simulink model "RADTRANS001"  (R2020b)
(part 2 of 6)

  Трансформатор_110_6_Район_{1..5} (5 alike) : powerlib/Elements/Three-Phase Transformer (Two Windings)  Winding1Connection=Yg  Winding2Connection=Yg  CoreType=Three single-phase transformers  SetSaturation=off  Hysteresis=off  DataFile='hysteresis'  SetInitialFlux=off  Measurements=None  UNITS=pu  NominalPower=[Tr_110_6_Sn_VA, Sys_f_Hz]  Winding1=[Tr_110_6_V_HV_kV*1e3, Tr_110_6_R_pu, Tr_110_6_L_pu]  Winding2=[Tr_110_6_V_LV_kV*1e3, Tr_110_6_R_pu, Tr_110_6_L_pu]  Rm=500  Lm=500  L0=0.5  Saturation=[ 0,0 ; 0.0024,1.2 ; 1.0,1.52 ]  InitialFluxes=[ 0.8 , -0.8 , 0.7 ]  BreakLoop=off  DiscreteSolver=Trapezoidal iterative  DataType=off  TransfoNumber=1
  Трансформатор_Город_1_{1..4} (4 alike) : powerlib/Elements/Three-Phase Transformer (Two Windings)  Winding1Connection=Yg  Winding2Connection=Yg  CoreType=Three single-phase transformers  SetSaturation=off  Hysteresis=off  DataFile='hysteresis'  SetInitialFlux=off  Measurements=None  UNITS=pu  NominalPower=[Tr_6_04_Sn_VA, Sys_f_Hz]  Winding1=[Tr_6_04_V_HV_kV*1e3, Tr_6_04_R_pu, Tr_6_04_L_pu]  Winding2=[Tr_6_04_V_LV_kV*1e3, Tr_6_04_R_pu, Tr_6_04_L_pu]  Rm=500  Lm=500  L0=0.5  Saturation=[ 0,0 ; 0.0024,1.2 ; 1.0,1.52 ]  InitialFluxes=[ 0.8 , -0.8 , 0.7 ]  BreakLoop=off  DiscreteSolver=Trapezoidal iterative  DataType=off  TransfoNumber=1
  Трансформатор_Город_2_{1..4} (4 alike) : powerlib/Elements/Three-Phase Transformer (Two Windings)  Winding1Connection=Yg  Winding2Connection=Yg  CoreType=Three single-phase transformers  SetSaturation=off  Hysteresis=off  DataFile='hysteresis'  SetInitialFlux=off  Measurements=None  UNITS=pu  NominalPower=[Tr_6_04_Sn_VA, Sys_f_Hz]  Winding1=[Tr_6_04_V_HV_kV*1e3, Tr_6_04_R_pu, Tr_6_04_L_pu]  Winding2=[Tr_6_04_V_LV_kV*1e3, Tr_6_04_R_pu, Tr_6_04_L_pu]  Rm=500  Lm=500  L0=0.5  Saturation=[ 0,0 ; 0.0024,1.2 ; 1.0,1.52 ]  InitialFluxes=[ 0.8 , -0.8 , 0.7 ]  BreakLoop=off  DiscreteSolver=Trapezoidal iterative  DataType=off  TransfoNumber=1
  Трансформатор_Город_3_{1..4} (4 alike) : powerlib/Elements/Three-Phase Transformer (Two Windings)  Winding1Connection=Yg  Winding2Connection=Yg  CoreType=Three single-phase transformers  SetSaturation=off  Hysteresis=off  DataFile='hysteresis'  SetInitialFlux=off  Measurements=None  UNITS=pu  NominalPower=[Tr_6_04_Sn_VA, Sys_f_Hz]  Winding1=[Tr_6_04_V_HV_kV*1e3, Tr_6_04_R_pu, Tr_6_04_L_pu]  Winding2=[Tr_6_04_V_LV_kV*1e3, Tr_6_04_R_pu, Tr_6_04_L_pu]  Rm=500  Lm=500  L0=0.5  Saturation=[ 0,0 ; 0.0024,1.2 ; 1.0,1.52 ]  InitialFluxes=[ 0.8 , -0.8 , 0.7 ]  BreakLoop=off  DiscreteSolver=Trapezoidal iterative  DataType=off  TransfoNumber=1
  Трансформатор_Город_4_{1..4} (4 alike) : powerlib/Elements/Three-Phase Transformer (Two Windings)  Winding1Connection=Yg  Winding2Connection=Yg  CoreType=Three single-phase transformers  SetSaturation=off  Hysteresis=off  DataFile='hysteresis'  SetInitialFlux=off  Measurements=None  UNITS=pu  NominalPower=[Tr_6_04_Sn_VA, Sys_f_Hz]  Winding1=[Tr_6_04_V_HV_kV*1e3, Tr_6_04_R_pu, Tr_6_04_L_pu]  Winding2=[Tr_6_04_V_LV_kV*1e3, Tr_6_04_R_pu, Tr_6_04_L_pu]  Rm=500  Lm=500  L0=0.5  Saturation=[ 0,0 ; 0.0024,1.2 ; 1.0,1.52 ]  InitialFluxes=[ 0.8 , -0.8 , 0.7 ]  BreakLoop=off  DiscreteSolver=Trapezoidal iterative  DataType=off  TransfoNumber=1
  Трансформатор_Город_5_{1..4} (4 alike) : powerlib/Elements/Three-Phase Transformer (Two Windings)  Winding1Connection=Yg  Winding2Connection=Yg  CoreType=Three single-phase transformers  SetSaturation=off  Hysteresis=off  DataFile='hysteresis'  SetInitialFlux=off  Measurements=None  UNITS=pu  NominalPower=[Tr_6_04_Sn_VA, Sys_f_Hz]  Winding1=[Tr_6_04_V_HV_kV*1e3, Tr_6_04_R_pu, Tr_6_04_L_pu]  Winding2=[Tr_6_04_V_LV_kV*1e3, Tr_6_04_R_pu, Tr_6_04_L_pu]  Rm=500  Lm=500  L0=0.5  Saturation=[ 0,0 ; 0.0024,1.2 ; 1.0,1.52 ]  InitialFluxes=[ 0.8 , -0.8 , 0.7 ]  BreakLoop=off  DiscreteSolver=Trapezoidal iterative  DataType=off  TransfoNumber=1
  Трансформатор_Завод_1_1 : powerlib/Elements/Three-Phase Transformer (Two Windings)  Winding1Connection=Yg  Winding2Connection=Yg  CoreType=Three single-phase transformers  SetSaturation=off  Hysteresis=off  DataFile='hysteresis'  SetInitialFlux=off  Measurements=None  UNITS=pu  NominalPower=[Tr_35_04_Sn_VA, Sys_f_Hz]  Winding1=[Tr_35_04_V_HV_kV*1e3, Tr_35_04_R_pu, Tr_35_04_L_pu]  Winding2=[Tr_35_04_V_LV_kV*1e3, Tr_35_04_R_pu, Tr_35_04_L_pu]  Rm=500  Lm=500  L0=0.5  Saturation=[ 0,0 ; 0.0024,1.2 ; 1.0,1.52 ]  InitialFluxes=[ 0.8 , -0.8 , 0.7 ]  BreakLoop=off  DiscreteSolver=Trapezoidal iterative  DataType=off  TransfoNumber=1
  Трансформатор_Завод_1_2 : powerlib/Elements/Three-Phase Transformer (Two Windings)  Winding1Connection=Yg  Winding2Connection=Yg  CoreType=Three single-phase transformers  SetSaturation=off  Hysteresis=off  DataFile='hysteresis'  SetInitialFlux=off  Measurements=None  UNITS=pu  NominalPower=[Tr_35_04_Sn_VA, Sys_f_Hz]  Winding1=[Tr_35_04_V_HV_kV*1e3, Tr_35_04_R_pu, Tr_35_04_L_pu]  Winding2=[Tr_35_04_V_LV_kV*1e3, Tr_35_04_R_pu, Tr_35_04_L_pu]  Rm=500  Lm=500  L0=0.5  Saturation=[ 0,0 ; 0.0024,1.2 ; 1.0,1.52 ]  InitialFluxes=[ 0.8 , -0.8 , 0.7 ]  BreakLoop=off  DiscreteSolver=Trapezoidal iterative  DataType=off  TransfoNumber=1
  Трансформатор_Завод_2_1 : powerlib/Elements/Three-Phase Transformer (Two Windings)  Winding1Connection=Yg  Winding2Connection=Yg  CoreType=Three single-phase transformers  SetSaturation=off  Hysteresis=off  DataFile='hysteresis'  SetInitialFlux=off  Measurements=None  UNITS=pu  NominalPower=[Tr_35_04_Sn_VA, Sys_f_Hz]  Winding1=[Tr_35_04_V_HV_kV*1e3, Tr_35_04_R_pu, Tr_35_04_L_pu]  Winding2=[Tr_35_04_V_LV_kV*1e3, Tr_35_04_R_pu, Tr_35_04_L_pu]  Rm=500  Lm=500  L0=0.5  Saturation=[ 0,0 ; 0.0024,1.2 ; 1.0,1.52 ]  InitialFluxes=[ 0.8 , -0.8 , 0.7 ]  BreakLoop=off  DiscreteSolver=Trapezoidal iterative  DataType=off  TransfoNumber=1
  Трансформатор_Завод_2_2 : powerlib/Elements/Three-Phase Transformer (Two Windings)  Winding1Connection=Yg  Winding2Connection=Yg  CoreType=Three single-phase transformers  SetSaturation=off  Hysteresis=off  DataFile='hysteresis'  SetInitialFlux=off  Measurements=None  UNITS=pu  NominalPower=[Tr_35_04_Sn_VA, Sys_f_Hz]  Winding1=[Tr_35_04_V_HV_kV*1e3, Tr_35_04_R_pu, Tr_35_04_L_pu]  Winding2=[Tr_35_04_V_LV_kV*1e3, Tr_35_04_R_pu, Tr_35_04_L_pu]  Rm=500  Lm=500  L0=0.5  Saturation=[ 0,0 ; 0.0024,1.2 ; 1.0,1.52 ]  InitialFluxes=[ 0.8 , -0.8 , 0.7 ]  BreakLoop=off  DiscreteSolver=Trapezoidal iterative  DataType=off  TransfoNumber=1
  Трансформатор_Завод_3_1 : powerlib/Elements/Three-Phase Transformer (Two Windings)  Winding1Connection=Yg  Winding2Connection=Yg  CoreType=Three single-phase transformers  SetSaturation=off  Hysteresis=off  DataFile='hysteresis'  SetInitialFlux=off  Measurements=None  UNITS=pu  NominalPower=[Tr_35_04_Sn_VA, Sys_f_Hz]  Winding1=[Tr_35_04_V_HV_kV*1e3, Tr_35_04_R_pu, Tr_35_04_L_pu]  Winding2=[Tr_35_04_V_LV_kV*1e3, Tr_35_04_R_pu, Tr_35_04_L_pu]  Rm=500  Lm=500  L0=0.5  Saturation=[ 0,0 ; 0.0024,1.2 ; 1.0,1.52 ]  InitialFluxes=[ 0.8 , -0.8 , 0.7 ]  BreakLoop=off  DiscreteSolver=Trapezoidal iterative  DataType=off  TransfoNumber=1
  Трансформатор_Завод_3_2 : powerlib/Elements/Three-Phase Transformer (Two Windings)  Winding1Connection=Yg  Winding2Connection=Yg  CoreType=Three single-phase transformers  SetSaturation=off  Hysteresis=off  DataFile='hysteresis'  SetInitialFlux=off  Measurements=None  UNITS=pu  NominalPower=[Tr_35_04_Sn_VA, Sys_f_Hz]  Winding1=[Tr_35_04_V_HV_kV*1e3, Tr_35_04_R_pu, Tr_35_04_L_pu]  Winding2=[Tr_35_04_V_LV_kV*1e3, Tr_35_04_R_pu, Tr_35_04_L_pu]  Rm=500  Lm=500  L0=0.5  Saturation=[ 0,0 ; 0.0024,1.2 ; 1.0,1.52 ]  InitialFluxes=[ 0.8 , -0.8 , 0.7 ]  BreakLoop=off  DiscreteSolver=Trapezoidal iterative  DataType=off  TransfoNumber=1
  Трансформатор_Завод_4_1 : powerlib/Elements/Three-Phase Transformer (Two Windings)  Winding1Connection=Yg  Winding2Connection=Yg  CoreType=Three single-phase transformers  SetSaturation=off  Hysteresis=off  DataFile='hysteresis'  SetInitialFlux=off  Measurements=None  UNITS=pu  NominalPower=[Tr_35_04_Sn_VA, Sys_f_Hz]  Winding1=[Tr_35_04_V_HV_kV*1e3, Tr_35_04_R_pu, Tr_35_04_L_pu]  Winding2=[Tr_35_04_V_LV_kV*1e3, Tr_35_04_R_pu, Tr_35_04_L_pu]  Rm=500  Lm=500  L0=0.5  Saturation=[ 0,0 ; 0.0024,1.2 ; 1.0,1.52 ]  InitialFluxes=[ 0.8 , -0.8 , 0.7 ]  BreakLoop=off  DiscreteSolver=Trapezoidal iterative  DataType=off  TransfoNumber=1
  Трансформатор_Завод_4_2 : powerlib/Elements/Three-Phase Transformer (Two Windings)  Winding1Connection=Yg  Winding2Connection=Yg  CoreType=Three single-phase transformers  SetSaturation=off  Hysteresis=off  DataFile='hysteresis'  SetInitialFlux=off  Measurements=None  UNITS=pu  NominalPower=[Tr_35_04_Sn_VA, Sys_f_Hz]  Winding1=[Tr_35_04_V_HV_kV*1e3, Tr_35_04_R_pu, Tr_35_04_L_pu]  Winding2=[Tr_35_04_V_LV_kV*1e3, Tr_35_04_R_pu, Tr_35_04_L_pu]  Rm=500  Lm=500  L0=0.5  Saturation=[ 0,0 ; 0.0024,1.2 ; 1.0,1.52 ]  InitialFluxes=[ 0.8 , -0.8 , 0.7 ]  BreakLoop=off  DiscreteSolver=Trapezoidal iterative  DataType=off  TransfoNumber=1
  Трансформатор_Завод_5_1 : powerlib/Elements/Three-Phase Transformer (Two Windings)  Winding1Connection=Yg  Winding2Connection=Yg  CoreType=Three single-phase transformers  SetSaturation=off  Hysteresis=off  DataFile='hysteresis'  SetInitialFlux=off  Measurements=None  UNITS=pu  NominalPower=[Tr_35_04_Sn_VA, Sys_f_Hz]  Winding1=[Tr_35_04_V_HV_kV*1e3, Tr_35_04_R_pu, Tr_35_04_L_pu]  Winding2=[Tr_35_04_V_LV_kV*1e3, Tr_35_04_R_pu, Tr_35_04_L_pu]  Rm=500  Lm=500  L0=0.5  Saturation=[ 0,0 ; 0.0024,1.2 ; 1.0,1.52 ]  InitialFluxes=[ 0.8 , -0.8 , 0.7 ]  BreakLoop=off  DiscreteSolver=Trapezoidal iterative  DataType=off  TransfoNumber=1
  Трансформатор_Завод_5_2 : powerlib/Elements/Three-Phase Transformer (Two Windings)  Winding1Connection=Yg  Winding2Connection=Yg  CoreType=Three single-phase transformers  SetSaturation=off  Hysteresis=off  DataFile='hysteresis'  SetInitialFlux=off  Measurements=None  UNITS=pu  NominalPower=[Tr_35_04_Sn_VA, Sys_f_Hz]  Winding1=[Tr_35_04_V_HV_kV*1e3, Tr_35_04_R_pu, Tr_35_04_L_pu]  Winding2=[Tr_35_04_V_LV_kV*1e3, Tr_35_04_R_pu, Tr_35_04_L_pu]  Rm=500  Lm=500  L0=0.5  Saturation=[ 0,0 ; 0.0024,1.2 ; 1.0,1.52 ]  InitialFluxes=[ 0.8 , -0.8 , 0.7 ]  BreakLoop=off  DiscreteSolver=Trapezoidal iterative  DataType=off  TransfoNumber=1
  Трансформатор_УРП_220_110 : powerlib/Elements/Three-Phase Transformer (Two Windings)  Winding1Connection=Yg  Winding2Connection=Yg  CoreType=Three single-phase transformers  SetSaturation=off  Hysteresis=off  DataFile='hysteresis'  SetInitialFlux=off  Measurements=None  UNITS=pu  NominalPower=[Tr_220_110_Sn_VA, Sys_f_Hz]  Winding1=[Tr_220_110_V_HV_kV*1e3, Tr_220_110_R_pu, Tr_220_110_L_pu]  Winding2=[Tr_220_110_V_LV_kV*1e3, Tr_220_110_R_pu, Tr_220_110_L_pu]  Rm=500  Lm=500  L0=0.5  Saturation=[ 0,0 ; 0.0024,1.2 ; 1.0,1.52 ]  InitialFluxes=[ 0.8 , -0.8 , 0.7 ]  BreakLoop=off  DiscreteSolver=Trapezoidal iterative  DataType=off  TransfoNumber=1
  connections:
  Источник_220кВ/RConn1 -- Магистраль_220кВ/LConn1
  Источник_220кВ/RConn2 -- Магистраль_220кВ/LConn2
  Источник_220кВ/RConn3 -- Магистраль_220кВ/LConn3
  Магистраль_220кВ/RConn1 -- Трансформатор_УРП_220_110/LConn1
  Магистраль_220кВ/RConn2 -- Трансформатор_УРП_220_110/LConn2
  Магистраль_220кВ/RConn3 -- Трансформатор_УРП_220_110/LConn3
  Линия_110кВ_Район_1/LConn1 -- Трансформатор_УРП_220_110/RConn1 -- Линия_110кВ_Район_2/LConn1 -- Линия_110кВ_Район_3/LConn1 -- Линия_110кВ_Район_4/LConn1 -- Линия_110кВ_Район_5/LConn1
  Линия_110кВ_Район_1/LConn2 -- Трансформатор_УРП_220_110/RConn2 -- Линия_110кВ_Район_2/LConn2 -- Линия_110кВ_Район_3/LConn2 -- Линия_110кВ_Район_4/LConn2 -- Линия_110кВ_Район_5/LConn2
  Линия_110кВ_Район_1/LConn3 -- Трансформатор_УРП_220_110/RConn3 -- Линия_110кВ_Район_2/LConn3 -- Линия_110кВ_Район_3/LConn3 -- Линия_110кВ_Район_4/LConn3 -- Линия_110кВ_Район_5/LConn3
  Трансформатор_110_35_Район_1/LConn1 -- Линия_110кВ_Район_1/RConn1 -- Трансформатор_110_6_Район_1/LConn1
  Трансформатор_110_35_Район_1/LConn2 -- Линия_110кВ_Район_1/RConn2 -- Трансформатор_110_6_Район_1/LConn2
  Трансформатор_110_35_Район_1/LConn3 -- Линия_110кВ_Район_1/RConn3 -- Трансформатор_110_6_Район_1/LConn3
  Линия_Завод_1_1/LConn1 -- Трансформатор_110_35_Район_1/RConn1 -- Линия_Завод_1_2/LConn1
  Линия_Завод_1_1/LConn2 -- Трансформатор_110_35_Район_1/RConn2 -- Линия_Завод_1_2/LConn2
  Линия_Завод_1_1/LConn3 -- Трансформатор_110_35_Район_1/RConn3 -- Линия_Завод_1_2/LConn3
  Линия_Завод_1_1/RConn1 -- M_IN_Завод_1_1/LConn1
  Линия_Завод_1_1/RConn2 -- M_IN_Завод_1_1/LConn2
  Линия_Завод_1_1/RConn3 -- M_IN_Завод_1_1/LConn3
  M_IN_Завод_1_1/RConn1 -- Трансформатор_Завод_1_1/LConn1
  M_IN_Завод_1_1/RConn2 -- Трансформатор_Завод_1_1/LConn2
  M_IN_Завод_1_1/RConn3 -- Трансформатор_Завод_1_1/LConn3
  Трансформатор_Завод_1_1/RConn1 -- M_OUT_Завод_1_1/LConn1
  Трансформатор_Завод_1_1/RConn2 -- M_OUT_Завод_1_1/LConn2
  Трансформатор_Завод_1_1/RConn3 -- M_OUT_Завод_1_1/LConn3
  M_OUT_Завод_1_1/RConn1 -- Нагрузка_Завод_1_1/LConn1
  M_OUT_Завод_1_1/RConn2 -- Нагрузка_Завод_1_1/LConn2
  M_OUT_Завод_1_1/RConn3 -- Нагрузка_Завод_1_1/LConn3
  Линия_Завод_1_2/RConn1 -- M_IN_Завод_1_2/LConn1
  Линия_Завод_1_2/RConn2 -- M_IN_Завод_1_2/LConn2
  Линия_Завод_1_2/RConn3 -- M_IN_Завод_1_2/LConn3
  M_IN_Завод_1_2/RConn1 -- Трансформатор_Завод_1_2/LConn1
  M_IN_Завод_1_2/RConn2 -- Трансформатор_Завод_1_2/LConn2
  M_IN_Завод_1_2/RConn3 -- Трансформатор_Завод_1_2/LConn3
  Трансформатор_Завод_1_2/RConn1 -- M_OUT_Завод_1_2/LConn1
  Трансформатор_Завод_1_2/RConn2 -- M_OUT_Завод_1_2/LConn2
  Трансформатор_Завод_1_2/RConn3 -- M_OUT_Завод_1_2/LConn3
  M_OUT_Завод_1_2/RConn1 -- Нагрузка_Завод_1_2/LConn1
  M_OUT_Завод_1_2/RConn2 -- Нагрузка_Завод_1_2/LConn2
  M_OUT_Завод_1_2/RConn3 -- Нагрузка_Завод_1_2/LConn3
  Линия_Город_1_1/LConn1 -- Трансформатор_110_6_Район_1/RConn1 -- Линия_Город_1_2/LConn1 -- Линия_Город_1_3/LConn1 -- Линия_Город_1_4/LConn1
  Линия_Город_1_1/LConn2 -- Трансформатор_110_6_Район_1/RConn2 -- Линия_Город_1_2/LConn2 -- Линия_Город_1_3/LConn2 -- Линия_Город_1_4/LConn2
  Линия_Город_1_1/LConn3 -- Трансформатор_110_6_Район_1/RConn3 -- Линия_Город_1_2/LConn3 -- Линия_Город_1_3/LConn3 -- Линия_Город_1_4/LConn3
  Линия_Город_1_1/RConn1 -- M_IN_Город_1_1/LConn1
  Линия_Город_1_1/RConn2 -- M_IN_Город_1_1/LConn2
  Линия_Город_1_1/RConn3 -- M_IN_Город_1_1/LConn3
  M_IN_Город_1_1/RConn1 -- Трансформатор_Город_1_1/LConn1
  M_IN_Город_1_1/RConn2 -- Трансформатор_Город_1_1/LConn2
  M_IN_Город_1_1/RConn3 -- Трансформатор_Город_1_1/LConn3
  Трансформатор_Город_1_1/RConn1 -- M_OUT_Город_1_1/LConn1
  Трансформатор_Город_1_1/RConn2 -- M_OUT_Город_1_1/LConn2
  Трансформатор_Город_1_1/RConn3 -- M_OUT_Город_1_1/LConn3
  M_OUT_Город_1_1/RConn1 -- Нагрузка_Город_1_1/LConn1
  M_OUT_Город_1_1/RConn2 -- Нагрузка_Город_1_1/LConn2
  M_OUT_Город_1_1/RConn3 -- Нагрузка_Город_1_1/LConn3
  Линия_Город_1_2/RConn1 -- M_IN_Город_1_2/LConn1
  Линия_Город_1_2/RConn2 -- M_IN_Город_1_2/LConn2
  Линия_Город_1_2/RConn3 -- M_IN_Город_1_2/LConn3
  M_IN_Город_1_2/RConn1 -- Трансформатор_Город_1_2/LConn1
  M_IN_Город_1_2/RConn2 -- Трансформатор_Город_1_2/LConn2
  M_IN_Город_1_2/RConn3 -- Трансформатор_Город_1_2/LConn3
  Трансформатор_Город_1_2/RConn1 -- M_OUT_Город_1_2/LConn1
  Трансформатор_Город_1_2/RConn2 -- M_OUT_Город_1_2/LConn2
  Трансформатор_Город_1_2/RConn3 -- M_OUT_Город_1_2/LConn3
  M_OUT_Город_1_2/RConn1 -- Нагрузка_Город_1_2/LConn1
  M_OUT_Город_1_2/RConn2 -- Нагрузка_Город_1_2/LConn2
  M_OUT_Город_1_2/RConn3 -- Нагрузка_Город_1_2/LConn3
  Линия_Город_1_3/RConn1 -- M_IN_Город_1_3/LConn1
  Линия_Город_1_3/RConn2 -- M_IN_Город_1_3/LConn2
  Линия_Город_1_3/RConn3 -- M_IN_Город_1_3/LConn3
  M_IN_Город_1_3/RConn1 -- Трансформатор_Город_1_3/LConn1
  M_IN_Город_1_3/RConn2 -- Трансформатор_Город_1_3/LConn2
  M_IN_Город_1_3/RConn3 -- Трансформатор_Город_1_3/LConn3
  Трансформатор_Город_1_3/RConn1 -- M_OUT_Город_1_3/LConn1
  Трансформатор_Город_1_3/RConn2 -- M_OUT_Город_1_3/LConn2
  Трансформатор_Город_1_3/RConn3 -- M_OUT_Город_1_3/LConn3
  M_OUT_Город_1_3/RConn1 -- Нагрузка_Город_1_3/LConn1
  M_OUT_Город_1_3/RConn2 -- Нагрузка_Город_1_3/LConn2
  M_OUT_Город_1_3/RConn3 -- Нагрузка_Город_1_3/LConn3
  Линия_Город_1_4/RConn1 -- M_IN_Город_1_4/LConn1
  Линия_Город_1_4/RConn2 -- M_IN_Город_1_4/LConn2
  Линия_Город_1_4/RConn3 -- M_IN_Город_1_4/LConn3
  M_IN_Город_1_4/RConn1 -- Трансформатор_Город_1_4/LConn1
  M_IN_Город_1_4/RConn2 -- Трансформатор_Город_1_4/LConn2
  M_IN_Город_1_4/RConn3 -- Трансформатор_Город_1_4/LConn3
  Трансформатор_Город_1_4/RConn1 -- M_OUT_Город_1_4/LConn1
  Трансформатор_Город_1_4/RConn2 -- M_OUT_Город_1_4/LConn2
  Трансформатор_Город_1_4/RConn3 -- M_OUT_Город_1_4/LConn3
  M_OUT_Город_1_4/RConn1 -- Нагрузка_Город_1_4/LConn1
  M_OUT_Город_1_4/RConn2 -- Нагрузка_Город_1_4/LConn2
  M_OUT_Город_1_4/RConn3 -- Нагрузка_Город_1_4/LConn3
  Трансформатор_110_35_Район_2/LConn1 -- Линия_110кВ_Район_2/RConn1 -- Трансформатор_110_6_Район_2/LConn1
  Трансформатор_110_35_Район_2/LConn2 -- Линия_110кВ_Район_2/RConn2 -- Трансформатор_110_6_Район_2/LConn2
  Трансформатор_110_35_Район_2/LConn3 -- Линия_110кВ_Район_2/RConn3 -- Трансформатор_110_6_Район_2/LConn3
  Линия_Завод_2_1/LConn1 -- Трансформатор_110_35_Район_2/RConn1 -- Линия_Завод_2_2/LConn1
  Линия_Завод_2_1/LConn2 -- Трансформатор_110_35_Район_2/RConn2 -- Линия_Завод_2_2/LConn2
  Линия_Завод_2_1/LConn3 -- Трансформатор_110_35_Район_2/RConn3 -- Линия_Завод_2_2/LConn3
  Линия_Завод_2_1/RConn1 -- M_IN_Завод_2_1/LConn1
  Линия_Завод_2_1/RConn2 -- M_IN_Завод_2_1/LConn2
  Линия_Завод_2_1/RConn3 -- M_IN_Завод_2_1/LConn3
  M_IN_Завод_2_1/RConn1 -- Трансформатор_Завод_2_1/LConn1
  M_IN_Завод_2_1/RConn2 -- Трансформатор_Завод_2_1/LConn2
  M_IN_Завод_2_1/RConn3 -- Трансформатор_Завод_2_1/LConn3
  Трансформатор_Завод_2_1/RConn1 -- M_OUT_Завод_2_1/LConn1
  Трансформатор_Завод_2_1/RConn2 -- M_OUT_Завод_2_1/LConn2
  Трансформатор_Завод_2_1/RConn3 -- M_OUT_Завод_2_1/LConn3
  M_OUT_Завод_2_1/RConn1 -- Нагрузка_Завод_2_1/LConn1
  M_OUT_Завод_2_1/RConn2 -- Нагрузка_Завод_2_1/LConn2
  M_OUT_Завод_2_1/RConn3 -- Нагрузка_Завод_2_1/LConn3
  Линия_Завод_2_2/RConn1 -- M_IN_Завод_2_2/LConn1
  Линия_Завод_2_2/RConn2 -- M_IN_Завод_2_2/LConn2
  Линия_Завод_2_2/RConn3 -- M_IN_Завод_2_2/LConn3
  M_IN_Завод_2_2/RConn1 -- Трансформатор_Завод_2_2/LConn1
  M_IN_Завод_2_2/RConn2 -- Трансформатор_Завод_2_2/LConn2
  M_IN_Завод_2_2/RConn3 -- Трансформатор_Завод_2_2/LConn3
  Трансформатор_Завод_2_2/RConn1 -- M_OUT_Завод_2_2/LConn1
  Трансформатор_Завод_2_2/RConn2 -- M_OUT_Завод_2_2/LConn2
  Трансформатор_Завод_2_2/RConn3 -- M_OUT_Завод_2_2/LConn3
  M_OUT_Завод_2_2/RConn1 -- Нагрузка_Завод_2_2/LConn1
  M_OUT_Завод_2_2/RConn2 -- Нагрузка_Завод_2_2/LConn2
  M_OUT_Завод_2_2/RConn3 -- Нагрузка_Завод_2_2/LConn3
  Линия_Город_2_1/LConn1 -- Трансформатор_110_6_Район_2/RConn1 -- Линия_Город_2_2/LConn1 -- Линия_Город_2_3/LConn1 -- Линия_Город_2_4/LConn1
  Линия_Город_2_1/LConn2 -- Трансформатор_110_6_Район_2/RConn2 -- Линия_Город_2_2/LConn2 -- Линия_Город_2_3/LConn2 -- Линия_Город_2_4/LConn2
  Линия_Город_2_1/LConn3 -- Трансформатор_110_6_Район_2/RConn3 -- Линия_Город_2_2/LConn3 -- Линия_Город_2_3/LConn3 -- Линия_Город_2_4/LConn3
  Линия_Город_2_1/RConn1 -- M_IN_Город_2_1/LConn1
  Линия_Город_2_1/RConn2 -- M_IN_Город_2_1/LConn2
  Линия_Город_2_1/RConn3 -- M_IN_Город_2_1/LConn3
  M_IN_Город_2_1/RConn1 -- Трансформатор_Город_2_1/LConn1
  M_IN_Город_2_1/RConn2 -- Трансформатор_Город_2_1/LConn2
  M_IN_Город_2_1/RConn3 -- Трансформатор_Город_2_1/LConn3
  Трансформатор_Город_2_1/RConn1 -- M_OUT_Город_2_1/LConn1
  Трансформатор_Город_2_1/RConn2 -- M_OUT_Город_2_1/LConn2
  Трансформатор_Город_2_1/RConn3 -- M_OUT_Город_2_1/LConn3
  M_OUT_Город_2_1/RConn1 -- Нагрузка_Город_2_1/LConn1
  M_OUT_Город_2_1/RConn2 -- Нагрузка_Город_2_1/LConn2
  M_OUT_Город_2_1/RConn3 -- Нагрузка_Город_2_1/LConn3
  Линия_Город_2_2/RConn1 -- M_IN_Город_2_2/LConn1
  Линия_Город_2_2/RConn2 -- M_IN_Город_2_2/LConn2
  Линия_Город_2_2/RConn3 -- M_IN_Город_2_2/LConn3
  M_IN_Город_2_2/RConn1 -- Трансформатор_Город_2_2/LConn1
  M_IN_Город_2_2/RConn2 -- Трансформатор_Город_2_2/LConn2
  M_IN_Город_2_2/RConn3 -- Трансформатор_Город_2_2/LConn3
  Трансформатор_Город_2_2/RConn1 -- M_OUT_Город_2_2/LConn1
  Трансформатор_Город_2_2/RConn2 -- M_OUT_Город_2_2/LConn2
  Трансформатор_Город_2_2/RConn3 -- M_OUT_Город_2_2/LConn3
  M_OUT_Город_2_2/RConn1 -- Нагрузка_Город_2_2/LConn1
  M_OUT_Город_2_2/RConn2 -- Нагрузка_Город_2_2/LConn2
  M_OUT_Город_2_2/RConn3 -- Нагрузка_Город_2_2/LConn3
  Линия_Город_2_3/RConn1 -- M_IN_Город_2_3/LConn1
  Линия_Город_2_3/RConn2 -- M_IN_Город_2_3/LConn2
  Линия_Город_2_3/RConn3 -- M_IN_Город_2_3/LConn3
  M_IN_Город_2_3/RConn1 -- Трансформатор_Город_2_3/LConn1
  M_IN_Город_2_3/RConn2 -- Трансформатор_Город_2_3/LConn2
  M_IN_Город_2_3/RConn3 -- Трансформатор_Город_2_3/LConn3
  Трансформатор_Город_2_3/RConn1 -- M_OUT_Город_2_3/LConn1
  Трансформатор_Город_2_3/RConn2 -- M_OUT_Город_2_3/LConn2
  Трансформатор_Город_2_3/RConn3 -- M_OUT_Город_2_3/LConn3
  M_OUT_Город_2_3/RConn1 -- Нагрузка_Город_2_3/LConn1
  M_OUT_Город_2_3/RConn2 -- Нагрузка_Город_2_3/LConn2
  M_OUT_Город_2_3/RConn3 -- Нагрузка_Город_2_3/LConn3
  Линия_Город_2_4/RConn1 -- M_IN_Город_2_4/LConn1
  Линия_Город_2_4/RConn2 -- M_IN_Город_2_4/LConn2
  Линия_Город_2_4/RConn3 -- M_IN_Город_2_4/LConn3
  M_IN_Город_2_4/RConn1 -- Трансформатор_Город_2_4/LConn1
  M_IN_Город_2_4/RConn2 -- Трансформатор_Город_2_4/LConn2
  M_IN_Город_2_4/RConn3 -- Трансформатор_Город_2_4/LConn3
  Трансформатор_Город_2_4/RConn1 -- M_OUT_Город_2_4/LConn1
  Трансформатор_Город_2_4/RConn2 -- M_OUT_Город_2_4/LConn2
  Трансформатор_Город_2_4/RConn3 -- M_OUT_Город_2_4/LConn3
  M_OUT_Город_2_4/RConn1 -- Нагрузка_Город_2_4/LConn1
  M_OUT_Город_2_4/RConn2 -- Нагрузка_Город_2_4/LConn2
  M_OUT_Город_2_4/RConn3 -- Нагрузка_Город_2_4/LConn3
  Трансформатор_110_35_Район_3/LConn1 -- Линия_110кВ_Район_3/RConn1 -- Трансформатор_110_6_Район_3/LConn1
  Трансформатор_110_35_Район_3/LConn2 -- Линия_110кВ_Район_3/RConn2 -- Трансформатор_110_6_Район_3/LConn2
  Трансформатор_110_35_Район_3/LConn3 -- Линия_110кВ_Район_3/RConn3 -- Трансформатор_110_6_Район_3/LConn3
  Линия_Завод_3_1/LConn1 -- Трансформатор_110_35_Район_3/RConn1 -- Линия_Завод_3_2/LConn1
  Линия_Завод_3_1/LConn2 -- Трансформатор_110_35_Район_3/RConn2 -- Линия_Завод_3_2/LConn2
  Линия_Завод_3_1/LConn3 -- Трансформатор_110_35_Район_3/RConn3 -- Линия_Завод_3_2/LConn3
  Линия_Завод_3_1/RConn1 -- M_IN_Завод_3_1/LConn1
  Линия_Завод_3_1/RConn2 -- M_IN_Завод_3_1/LConn2
  Линия_Завод_3_1/RConn3 -- M_IN_Завод_3_1/LConn3
  M_IN_Завод_3_1/RConn1 -- Трансформатор_Завод_3_1/LConn1
  M_IN_Завод_3_1/RConn2 -- Трансформатор_Завод_3_1/LConn2
  M_IN_Завод_3_1/RConn3 -- Трансформатор_Завод_3_1/LConn3
  Трансформатор_Завод_3_1/RConn1 -- M_OUT_Завод_3_1/LConn1
  Трансформатор_Завод_3_1/RConn2 -- M_OUT_Завод_3_1/LConn2
  Трансформатор_Завод_3_1/RConn3 -- M_OUT_Завод_3_1/LConn3
  M_OUT_Завод_3_1/RConn1 -- Нагрузка_Завод_3_1/LConn1
  M_OUT_Завод_3_1/RConn2 -- Нагрузка_Завод_3_1/LConn2
  M_OUT_Завод_3_1/RConn3 -- Нагрузка_Завод_3_1/LConn3
  Линия_Завод_3_2/RConn1 -- M_IN_Завод_3_2/LConn1
  Линия_Завод_3_2/RConn2 -- M_IN_Завод_3_2/LConn2
  Линия_Завод_3_2/RConn3 -- M_IN_Завод_3_2/LConn3
  M_IN_Завод_3_2/RConn1 -- Трансформатор_Завод_3_2/LConn1
  M_IN_Завод_3_2/RConn2 -- Трансформатор_Завод_3_2/LConn2
  M_IN_Завод_3_2/RConn3 -- Трансформатор_Завод_3_2/LConn3
  Трансформатор_Завод_3_2/RConn1 -- M_OUT_Завод_3_2/LConn1
  Трансформатор_Завод_3_2/RConn2 -- M_OUT_Завод_3_2/LConn2
  Трансформатор_Завод_3_2/RConn3 -- M_OUT_Завод_3_2/LConn3
  M_OUT_Завод_3_2/RConn1 -- Нагрузка_Завод_3_2/LConn1
  M_OUT_Завод_3_2/RConn2 -- Нагрузка_Завод_3_2/LConn2
  M_OUT_Завод_3_2/RConn3 -- Нагрузка_Завод_3_2/LConn3
  Линия_Город_3_1/LConn1 -- Трансформатор_110_6_Район_3/RConn1 -- Линия_Город_3_2/LConn1 -- Линия_Город_3_3/LConn1 -- Линия_Город_3_4/LConn1
  Линия_Город_3_1/LConn2 -- Трансформатор_110_6_Район_3/RConn2 -- Линия_Город_3_2/LConn2 -- Линия_Город_3_3/LConn2 -- Линия_Город_3_4/LConn2
  Линия_Город_3_1/LConn3 -- Трансформатор_110_6_Район_3/RConn3 -- Линия_Город_3_2/LConn3 -- Линия_Город_3_3/LConn3 -- Линия_Город_3_4/LConn3
  Линия_Город_3_1/RConn1 -- M_IN_Город_3_1/LConn1
  Линия_Город_3_1/RConn2 -- M_IN_Город_3_1/LConn2
  Линия_Город_3_1/RConn3 -- M_IN_Город_3_1/LConn3
  M_IN_Город_3_1/RConn1 -- Трансформатор_Город_3_1/LConn1
  M_IN_Город_3_1/RConn2 -- Трансформатор_Город_3_1/LConn2
  M_IN_Город_3_1/RConn3 -- Трансформатор_Город_3_1/LConn3
  Трансформатор_Город_3_1/RConn1 -- M_OUT_Город_3_1/LConn1
  Трансформатор_Город_3_1/RConn2 -- M_OUT_Город_3_1/LConn2
  Трансформатор_Город_3_1/RConn3 -- M_OUT_Город_3_1/LConn3
  M_OUT_Город_3_1/RConn1 -- Нагрузка_Город_3_1/LConn1
  M_OUT_Город_3_1/RConn2 -- Нагрузка_Город_3_1/LConn2
  M_OUT_Город_3_1/RConn3 -- Нагрузка_Город_3_1/LConn3
  Линия_Город_3_2/RConn1 -- M_IN_Город_3_2/LConn1
  Линия_Город_3_2/RConn2 -- M_IN_Город_3_2/LConn2
  Линия_Город_3_2/RConn3 -- M_IN_Город_3_2/LConn3
  M_IN_Город_3_2/RConn1 -- Трансформатор_Город_3_2/LConn1
  M_IN_Город_3_2/RConn2 -- Трансформатор_Город_3_2/LConn2
  M_IN_Город_3_2/RConn3 -- Трансформатор_Город_3_2/LConn3
  Трансформатор_Город_3_2/RConn1 -- M_OUT_Город_3_2/LConn1
  Трансформатор_Город_3_2/RConn2 -- M_OUT_Город_3_2/LConn2
  Трансформатор_Город_3_2/RConn3 -- M_OUT_Город_3_2/LConn3
  M_OUT_Город_3_2/RConn1 -- Нагрузка_Город_3_2/LConn1
  M_OUT_Город_3_2/RConn2 -- Нагрузка_Город_3_2/LConn2
  M_OUT_Город_3_2/RConn3 -- Нагрузка_Город_3_2/LConn3
  Линия_Город_3_3/RConn1 -- M_IN_Город_3_3/LConn1
  Линия_Город_3_3/RConn2 -- M_IN_Город_3_3/LConn2
  Линия_Город_3_3/RConn3 -- M_IN_Город_3_3/LConn3
  M_IN_Город_3_3/RConn1 -- Трансформатор_Город_3_3/LConn1
  M_IN_Город_3_3/RConn2 -- Трансформатор_Город_3_3/LConn2
  M_IN_Город_3_3/RConn3 -- Трансформатор_Город_3_3/LConn3
  Трансформатор_Город_3_3/RConn1 -- M_OUT_Город_3_3/LConn1
  Трансформатор_Город_3_3/RConn2 -- M_OUT_Город_3_3/LConn2
  Трансформатор_Город_3_3/RConn3 -- M_OUT_Город_3_3/LConn3
  M_OUT_Город_3_3/RConn1 -- Нагрузка_Город_3_3/LConn1
  M_OUT_Город_3_3/RConn2 -- Нагрузка_Город_3_3/LConn2
  M_OUT_Город_3_3/RConn3 -- Нагрузка_Город_3_3/LConn3
  Линия_Город_3_4/RConn1 -- M_IN_Город_3_4/LConn1
  Линия_Город_3_4/RConn2 -- M_IN_Город_3_4/LConn2
  Линия_Город_3_4/RConn3 -- M_IN_Город_3_4/LConn3
  M_IN_Город_3_4/RConn1 -- Трансформатор_Город_3_4/LConn1
  M_IN_Город_3_4/RConn2 -- Трансформатор_Город_3_4/LConn2
  M_IN_Город_3_4/RConn3 -- Трансформатор_Город_3_4/LConn3
  Трансформатор_Город_3_4/RConn1 -- M_OUT_Город_3_4/LConn1
  Трансформатор_Город_3_4/RConn2 -- M_OUT_Город_3_4/LConn2
  Трансформатор_Город_3_4/RConn3 -- M_OUT_Город_3_4/LConn3
  M_OUT_Город_3_4/RConn1 -- Нагрузка_Город_3_4/LConn1
  M_OUT_Город_3_4/RConn2 -- Нагрузка_Город_3_4/LConn2
  M_OUT_Город_3_4/RConn3 -- Нагрузка_Город_3_4/LConn3
  Трансформатор_110_35_Район_4/LConn1 -- Линия_110кВ_Район_4/RConn1 -- Трансформатор_110_6_Район_4/LConn1
  Трансформатор_110_35_Район_4/LConn2 -- Линия_110кВ_Район_4/RConn2 -- Трансформатор_110_6_Район_4/LConn2
  Трансформатор_110_35_Район_4/LConn3 -- Линия_110кВ_Район_4/RConn3 -- Трансформатор_110_6_Район_4/LConn3
  Линия_Завод_4_1/LConn1 -- Трансформатор_110_35_Район_4/RConn1 -- Линия_Завод_4_2/LConn1
  Линия_Завод_4_1/LConn2 -- Трансформатор_110_35_Район_4/RConn2 -- Линия_Завод_4_2/LConn2
  Линия_Завод_4_1/LConn3 -- Трансформатор_110_35_Район_4/RConn3 -- Линия_Завод_4_2/LConn3
  Линия_Завод_4_1/RConn1 -- M_IN_Завод_4_1/LConn1
  Линия_Завод_4_1/RConn2 -- M_IN_Завод_4_1/LConn2
  Линия_Завод_4_1/RConn3 -- M_IN_Завод_4_1/LConn3
  M_IN_Завод_4_1/RConn1 -- Трансформатор_Завод_4_1/LConn1
  M_IN_Завод_4_1/RConn2 -- Трансформатор_Завод_4_1/LConn2
  M_IN_Завод_4_1/RConn3 -- Трансформатор_Завод_4_1/LConn3
  Трансформатор_Завод_4_1/RConn1 -- M_OUT_Завод_4_1/LConn1
  Трансформатор_Завод_4_1/RConn2 -- M_OUT_Завод_4_1/LConn2
  Трансформатор_Завод_4_1/RConn3 -- M_OUT_Завод_4_1/LConn3
  M_OUT_Завод_4_1/RConn1 -- Нагрузка_Завод_4_1/LConn1
  M_OUT_Завод_4_1/RConn2 -- Нагрузка_Завод_4_1/LConn2
  M_OUT_Завод_4_1/RConn3 -- Нагрузка_Завод_4_1/LConn3
  Линия_Завод_4_2/RConn1 -- M_IN_Завод_4_2/LConn1
  Линия_Завод_4_2/RConn2 -- M_IN_Завод_4_2/LConn2
  Линия_Завод_4_2/RConn3 -- M_IN_Завод_4_2/LConn3
  M_IN_Завод_4_2/RConn1 -- Трансформатор_Завод_4_2/LConn1
  M_IN_Завод_4_2/RConn2 -- Трансформатор_Завод_4_2/LConn2
  M_IN_Завод_4_2/RConn3 -- Трансформатор_Завод_4_2/LConn3
  Трансформатор_Завод_4_2/RConn1 -- M_OUT_Завод_4_2/LConn1
  Трансформатор_Завод_4_2/RConn2 -- M_OUT_Завод_4_2/LConn2
  Трансформатор_Завод_4_2/RConn3 -- M_OUT_Завод_4_2/LConn3
  M_OUT_Завод_4_2/RConn1 -- Нагрузка_Завод_4_2/LConn1
  M_OUT_Завод_4_2/RConn2 -- Нагрузка_Завод_4_2/LConn2
  M_OUT_Завод_4_2/RConn3 -- Нагрузка_Завод_4_2/LConn3
  Линия_Город_4_1/LConn1 -- Трансформатор_110_6_Район_4/RConn1 -- Линия_Город_4_2/LConn1 -- Линия_Город_4_3/LConn1 -- Линия_Город_4_4/LConn1
  Линия_Город_4_1/LConn2 -- Трансформатор_110_6_Район_4/RConn2 -- Линия_Город_4_2/LConn2 -- Линия_Город_4_3/LConn2 -- Линия_Город_4_4/LConn2
  Линия_Город_4_1/LConn3 -- Трансформатор_110_6_Район_4/RConn3 -- Линия_Город_4_2/LConn3 -- Линия_Город_4_3/LConn3 -- Линия_Город_4_4/LConn3
  Линия_Город_4_1/RConn1 -- M_IN_Город_4_1/LConn1
  Линия_Город_4_1/RConn2 -- M_IN_Город_4_1/LConn2
  Линия_Город_4_1/RConn3 -- M_IN_Город_4_1/LConn3
  M_IN_Город_4_1/RConn1 -- Трансформатор_Город_4_1/LConn1
  M_IN_Город_4_1/RConn2 -- Трансформатор_Город_4_1/LConn2
  M_IN_Город_4_1/RConn3 -- Трансформатор_Город_4_1/LConn3
  Трансформатор_Город_4_1/RConn1 -- M_OUT_Город_4_1/LConn1
  Трансформатор_Город_4_1/RConn2 -- M_OUT_Город_4_1/LConn2
  Трансформатор_Город_4_1/RConn3 -- M_OUT_Город_4_1/LConn3
  M_OUT_Город_4_1/RConn1 -- Нагрузка_Город_4_1/LConn1
  M_OUT_Город_4_1/RConn2 -- Нагрузка_Город_4_1/LConn2
  M_OUT_Город_4_1/RConn3 -- Нагрузка_Город_4_1/LConn3
  Линия_Город_4_2/RConn1 -- M_IN_Город_4_2/LConn1
  Линия_Город_4_2/RConn2 -- M_IN_Город_4_2/LConn2
  Линия_Город_4_2/RConn3 -- M_IN_Город_4_2/LConn3
  M_IN_Город_4_2/RConn1 -- Трансформатор_Город_4_2/LConn1
  M_IN_Город_4_2/RConn2 -- Трансформатор_Город_4_2/LConn2
  M_IN_Город_4_2/RConn3 -- Трансформатор_Город_4_2/LConn3
  Трансформатор_Город_4_2/RConn1 -- M_OUT_Город_4_2/LConn1
  Трансформатор_Город_4_2/RConn2 -- M_OUT_Город_4_2/LConn2
  Трансформатор_Город_4_2/RConn3 -- M_OUT_Город_4_2/LConn3
  M_OUT_Город_4_2/RConn1 -- Нагрузка_Город_4_2/LConn1
  M_OUT_Город_4_2/RConn2 -- Нагрузка_Город_4_2/LConn2
  M_OUT_Город_4_2/RConn3 -- Нагрузка_Город_4_2/LConn3
  Линия_Город_4_3/RConn1 -- M_IN_Город_4_3/LConn1
  Линия_Город_4_3/RConn2 -- M_IN_Город_4_3/LConn2
  Линия_Город_4_3/RConn3 -- M_IN_Город_4_3/LConn3
  M_IN_Город_4_3/RConn1 -- Трансформатор_Город_4_3/LConn1
  M_IN_Город_4_3/RConn2 -- Трансформатор_Город_4_3/LConn2
  M_IN_Город_4_3/RConn3 -- Трансформатор_Город_4_3/LConn3
  Трансформатор_Город_4_3/RConn1 -- M_OUT_Город_4_3/LConn1
  Трансформатор_Город_4_3/RConn2 -- M_OUT_Город_4_3/LConn2
  Трансформатор_Город_4_3/RConn3 -- M_OUT_Город_4_3/LConn3
  M_OUT_Город_4_3/RConn1 -- Нагрузка_Город_4_3/LConn1
  M_OUT_Город_4_3/RConn2 -- Нагрузка_Город_4_3/LConn2
  M_OUT_Город_4_3/RConn3 -- Нагрузка_Город_4_3/LConn3
  Линия_Город_4_4/RConn1 -- M_IN_Город_4_4/LConn1
  Линия_Город_4_4/RConn2 -- M_IN_Город_4_4/LConn2
  Линия_Город_4_4/RConn3 -- M_IN_Город_4_4/LConn3
  M_IN_Город_4_4/RConn1 -- Трансформатор_Город_4_4/LConn1
  M_IN_Город_4_4/RConn2 -- Трансформатор_Город_4_4/LConn2
  M_IN_Город_4_4/RConn3 -- Трансформатор_Город_4_4/LConn3
  Трансформатор_Город_4_4/RConn1 -- M_OUT_Город_4_4/LConn1
  Трансформатор_Город_4_4/RConn2 -- M_OUT_Город_4_4/LConn2
  Трансформатор_Город_4_4/RConn3 -- M_OUT_Город_4_4/LConn3
  M_OUT_Город_4_4/RConn1 -- Нагрузка_Город_4_4/LConn1
  M_OUT_Город_4_4/RConn2 -- Нагрузка_Город_4_4/LConn2
  M_OUT_Город_4_4/RConn3 -- Нагрузка_Город_4_4/LConn3
  Трансформатор_110_35_Район_5/LConn1 -- Линия_110кВ_Район_5/RConn1 -- Трансформатор_110_6_Район_5/LConn1
  Трансформатор_110_35_Район_5/LConn2 -- Линия_110кВ_Район_5/RConn2 -- Трансформатор_110_6_Район_5/LConn2
  Трансформатор_110_35_Район_5/LConn3 -- Линия_110кВ_Район_5/RConn3 -- Трансформатор_110_6_Район_5/LConn3
  Линия_Завод_5_1/LConn1 -- Трансформатор_110_35_Район_5/RConn1 -- Линия_Завод_5_2/LConn1
  Линия_Завод_5_1/LConn2 -- Трансформатор_110_35_Район_5/RConn2 -- Линия_Завод_5_2/LConn2
  Линия_Завод_5_1/LConn3 -- Трансформатор_110_35_Район_5/RConn3 -- Линия_Завод_5_2/LConn3
  Линия_Завод_5_1/RConn1 -- M_IN_Завод_5_1/LConn1
  Линия_Завод_5_1/RConn2 -- M_IN_Завод_5_1/LConn2
  Линия_Завод_5_1/RConn3 -- M_IN_Завод_5_1/LConn3
  M_IN_Завод_5_1/RConn1 -- Трансформатор_Завод_5_1/LConn1
  M_IN_Завод_5_1/RConn2 -- Трансформатор_Завод_5_1/LConn2
  M_IN_Завод_5_1/RConn3 -- Трансформатор_Завод_5_1/LConn3
  Трансформатор_Завод_5_1/RConn1 -- M_OUT_Завод_5_1/LConn1
  Трансформатор_Завод_5_1/RConn2 -- M_OUT_Завод_5_1/LConn2
  Трансформатор_Завод_5_1/RConn3 -- M_OUT_Завод_5_1/LConn3
  M_OUT_Завод_5_1/RConn1 -- Нагрузка_Завод_5_1/LConn1
  M_OUT_Завод_5_1/RConn2 -- Нагрузка_Завод_5_1/LConn2
  M_OUT_Завод_5_1/RConn3 -- Нагрузка_Завод_5_1/LConn3
  Линия_Завод_5_2/RConn1 -- M_IN_Завод_5_2/LConn1
  Линия_Завод_5_2/RConn2 -- M_IN_Завод_5_2/LConn2
  Линия_Завод_5_2/RConn3 -- M_IN_Завод_5_2/LConn3
  M_IN_Завод_5_2/RConn1 -- Трансформатор_Завод_5_2/LConn1
  M_IN_Завод_5_2/RConn2 -- Трансформатор_Завод_5_2/LConn2
  M_IN_Завод_5_2/RConn3 -- Трансформатор_Завод_5_2/LConn3
  Трансформатор_Завод_5_2/RConn1 -- M_OUT_Завод_5_2/LConn1
  Трансформатор_Завод_5_2/RConn2 -- M_OUT_Завод_5_2/LConn2
  Трансформатор_Завод_5_2/RConn3 -- M_OUT_Завод_5_2/LConn3
  M_OUT_Завод_5_2/RConn1 -- Нагрузка_Завод_5_2/LConn1
  M_OUT_Завод_5_2/RConn2 -- Нагрузка_Завод_5_2/LConn2
  M_OUT_Завод_5_2/RConn3 -- Нагрузка_Завод_5_2/LConn3
  Линия_Город_5_1/LConn1 -- Трансформатор_110_6_Район_5/RConn1 -- Линия_Город_5_2/LConn1 -- Линия_Город_5_3/LConn1 -- Линия_Город_5_4/LConn1
  Линия_Город_5_1/LConn2 -- Трансформатор_110_6_Район_5/RConn2 -- Линия_Город_5_2/LConn2 -- Линия_Город_5_3/LConn2 -- Линия_Город_5_4/LConn2
  Линия_Город_5_1/LConn3 -- Трансформатор_110_6_Район_5/RConn3 -- Линия_Город_5_2/LConn3 -- Линия_Город_5_3/LConn3 -- Линия_Город_5_4/LConn3
  Линия_Город_5_1/RConn1 -- M_IN_Город_5_1/LConn1
  Линия_Город_5_1/RConn2 -- M_IN_Город_5_1/LConn2
  Линия_Город_5_1/RConn3 -- M_IN_Город_5_1/LConn3
  M_IN_Город_5_1/RConn1 -- Трансформатор_Город_5_1/LConn1
  M_IN_Город_5_1/RConn2 -- Трансформатор_Город_5_1/LConn2
  M_IN_Город_5_1/RConn3 -- Трансформатор_Город_5_1/LConn3
  Трансформатор_Город_5_1/RConn1 -- M_OUT_Город_5_1/LConn1
  Трансформатор_Город_5_1/RConn2 -- M_OUT_Город_5_1/LConn2
  Трансформатор_Город_5_1/RConn3 -- M_OUT_Город_5_1/LConn3
  M_OUT_Город_5_1/RConn1 -- Нагрузка_Город_5_1/LConn1
  M_OUT_Город_5_1/RConn2 -- Нагрузка_Город_5_1/LConn2
  M_OUT_Город_5_1/RConn3 -- Нагрузка_Город_5_1/LConn3
  Линия_Город_5_2/RConn1 -- M_IN_Город_5_2/LConn1
  Линия_Город_5_2/RConn2 -- M_IN_Город_5_2/LConn2
  Линия_Город_5_2/RConn3 -- M_IN_Город_5_2/LConn3
  M_IN_Город_5_2/RConn1 -- Трансформатор_Город_5_2/LConn1
  M_IN_Город_5_2/RConn2 -- Трансформатор_Город_5_2/LConn2
  M_IN_Город_5_2/RConn3 -- Трансформатор_Город_5_2/LConn3
  Трансформатор_Город_5_2/RConn1 -- M_OUT_Город_5_2/LConn1
  Трансформатор_Город_5_2/RConn2 -- M_OUT_Город_5_2/LConn2
  Трансформатор_Город_5_2/RConn3 -- M_OUT_Город_5_2/LConn3
  M_OUT_Город_5_2/RConn1 -- Нагрузка_Город_5_2/LConn1
  M_OUT_Город_5_2/RConn2 -- Нагрузка_Город_5_2/LConn2
  M_OUT_Город_5_2/RConn3 -- Нагрузка_Город_5_2/LConn3
  Линия_Город_5_3/RConn1 -- M_IN_Город_5_3/LConn1
  Линия_Город_5_3/RConn2 -- M_IN_Город_5_3/LConn2
  Линия_Город_5_3/RConn3 -- M_IN_Город_5_3/LConn3
  M_IN_Город_5_3/RConn1 -- Трансформатор_Город_5_3/LConn1
  M_IN_Город_5_3/RConn2 -- Трансформатор_Город_5_3/LConn2
  M_IN_Город_5_3/RConn3 -- Трансформатор_Город_5_3/LConn3
  Трансформатор_Город_5_3/RConn1 -- M_OUT_Город_5_3/LConn1
  Трансформатор_Город_5_3/RConn2 -- M_OUT_Город_5_3/LConn2
  Трансформатор_Город_5_3/RConn3 -- M_OUT_Город_5_3/LConn3
  M_OUT_Город_5_3/RConn1 -- Нагрузка_Город_5_3/LConn1
  M_OUT_Город_5_3/RConn2 -- Нагрузка_Город_5_3/LConn2
  M_OUT_Город_5_3/RConn3 -- Нагрузка_Город_5_3/LConn3
  Линия_Город_5_4/RConn1 -- M_IN_Город_5_4/LConn1
  Линия_Город_5_4/RConn2 -- M_IN_Город_5_4/LConn2
  Линия_Город_5_4/RConn3 -- M_IN_Город_5_4/LConn3
  M_IN_Город_5_4/RConn1 -- Трансформатор_Город_5_4/LConn1
  M_IN_Город_5_4/RConn2 -- Трансформатор_Город_5_4/LConn2
  M_IN_Город_5_4/RConn3 -- Трансформатор_Город_5_4/LConn3
  Трансформатор_Город_5_4/RConn1 -- M_OUT_Город_5_4/LConn1
  Трансформатор_Город_5_4/RConn2 -- M_OUT_Город_5_4/LConn2
  Трансформатор_Город_5_4/RConn3 -- M_OUT_Город_5_4/LConn3
  M_OUT_Город_5_4/RConn1 -- Нагрузка_Город_5_4/LConn1
  M_OUT_Город_5_4/RConn2 -- Нагрузка_Город_5_4/LConn2
  M_OUT_Город_5_4/RConn3 -- Нагрузка_Город_5_4/LConn3
